simulink library "Sensors_Lib"  (R2018b)
settings: Solver=VariableStepAuto  StartTime=0.0  StopTime=10.0  RelTol=1e-3
undefined symbols (not defined in the file or in its folder): gyro_body_radps, gyro_meas_valid, mag_body_T, mag_meas_valid, photodiodes_A, solar_panel_power_W, sun_meas_ss_deg, sun_meas_valid
libraries: gyroscope_lib x3, magnetometer_lib x3, sensor_bus x1, solar_panels_lib x1, sun_sensor_lib x1
settings Model: Creator=colem  LastModifiedBy=Taylor

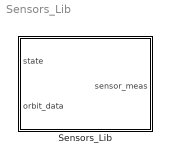
== system Sensors_Lib ==
  Sensors_Lib : Subsystem

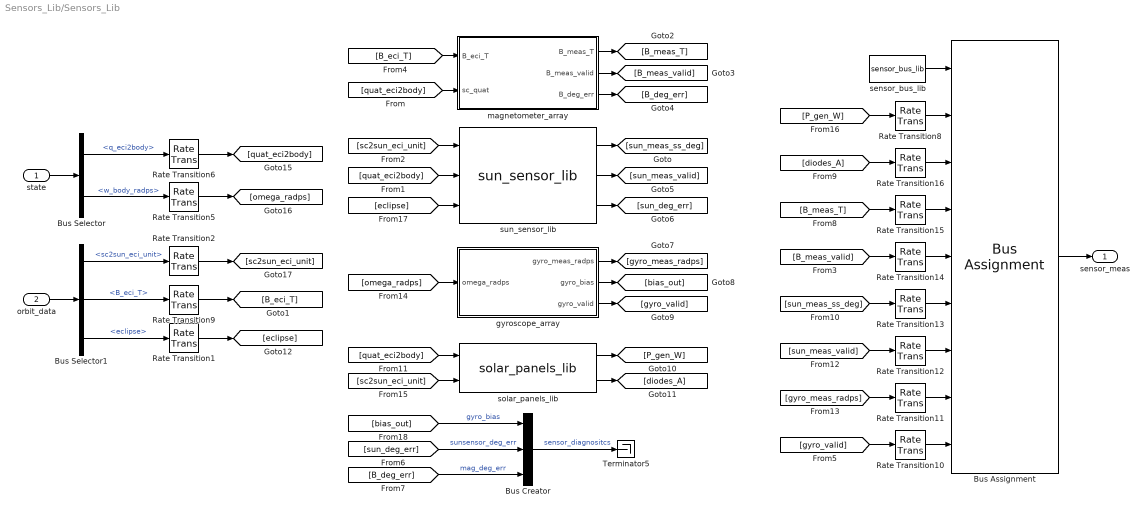
== system Sensors_Lib/Sensors_Lib ==
  state : Inport  OutDataTypeStr=Bus: state
  orbit_data : Inport  Port=2  OutDataTypeStr=Bus: orbit_data
  Bus Assignment : BusAssignment  AssignedSignals=solar_panel_power_W,photodiodes_A,mag_body_T,mag_meas_valid,sun_meas_ss_deg,sun_meas_valid,gyro_body_radps,gyro_meas_valid
  Bus Creator : BusCreator  Inputs=3
  Bus Selector : BusSelector  OutputSignals=q_eci2body,w_body_radps
  Bus Selector1 : BusSelector  OutputSignals=sc2sun_eci_unit,B_eci_T,eclipse
  Rate Transition{1..2,5..6,8..16} (13 alike) : RateTransition  OutPortSampleTime=simParams.sensors.sample_time_s
  Terminator5 : Terminator
  gyroscope_array : Subsystem
  magnetometer_array : Subsystem
  sensor_bus_lib : sensor_bus/sensor_bus_lib  SystemSampleTime=-1
  solar_panels_lib : solar_panels_lib/solar_panels_lib  SystemSampleTime=-1
  "sun_sensor_lib " : sun_sensor_lib/sun_sensor_lib   SystemSampleTime=-1
  sensor_meas : Outport  OutDataTypeStr=Bus: sensor_bus
  wires:
  Bus Selector/2 -> Rate Transition5/1  "<w_body_radps>"
  Bus Assignment/1 -> sensor_meas/1
  [quat_eci2body] -> magnetometer_array/2(sc_quat)
  [quat_eci2body] -> "sun_sensor_lib "/2
  [omega_radps] -> gyroscope_array/1(omega_radps)
  orbit_data/1 -> Bus Selector1/1
  [sc2sun_eci_unit] -> "sun_sensor_lib "/1
  [B_eci_T] -> magnetometer_array/1(B_eci_T)
  sensor_bus_lib/1 -> Bus Assignment/1
  magnetometer_array/1(B_meas_T) -> [B_meas_T]
  magnetometer_array/2(B_meas_valid) -> [B_meas_valid]
  magnetometer_array/3(B_deg_err) -> [B_deg_err]
  "sun_sensor_lib "/1 -> [sun_meas_ss_deg]
  "sun_sensor_lib "/2 -> [sun_meas_valid]
  "sun_sensor_lib "/3 -> [sun_deg_err]
  gyroscope_array/1(gyro_meas_radps) -> [gyro_meas_radps]
  gyroscope_array/2(gyro_bias) -> [bias_out]
  gyroscope_array/3(gyro_valid) -> [gyro_valid]
  Rate Transition5/1 -> [omega_radps]
  Bus Selector/1 -> Rate Transition6/1  "<q_eci2body>"
  Rate Transition6/1 -> [quat_eci2body]
  Bus Selector1/2 -> Rate Transition9/1  "<B_eci_T>"
  Rate Transition9/1 -> [B_eci_T]
  Bus Selector1/1 -> Rate Transition2/1  "<sc2sun_eci_unit>"
  Rate Transition2/1 -> [sc2sun_eci_unit]
  [sc2sun_eci_unit] -> solar_panels_lib/2
  [quat_eci2body] -> solar_panels_lib/1
  solar_panels_lib/1 -> [P_gen_W]
  [B_meas_T] -> Rate Transition15/1
  [P_gen_W] -> Rate Transition8/1
  [B_meas_valid] -> Rate Transition14/1
  [sun_meas_ss_deg] -> Rate Transition13/1
  [sun_meas_valid] -> Rate Transition12/1
  [gyro_meas_radps] -> Rate Transition11/1
  [gyro_valid] -> Rate Transition10/1
  [bias_out] -> Bus Creator/1  "gyro_bias"
  [sun_deg_err] -> Bus Creator/2  "sunsensor_deg_err"
  [B_deg_err] -> Bus Creator/3  "mag_deg_err"
  Bus Creator/1 -> Terminator5/1  "sensor_diagnositcs"
  solar_panels_lib/2 -> [diodes_A]
  Rate Transition10/1 -> Bus Assignment/9
  Rate Transition11/1 -> Bus Assignment/8
  Rate Transition12/1 -> Bus Assignment/7
  Rate Transition13/1 -> Bus Assignment/6
  Rate Transition14/1 -> Bus Assignment/5
  Rate Transition15/1 -> Bus Assignment/4
  Rate Transition8/1 -> Bus Assignment/2
  Rate Transition16/1 -> Bus Assignment/3
  [diodes_A] -> Rate Transition16/1
  state/1 -> Bus Selector/1
  Bus Selector1/3 -> Rate Transition1/1  "<eclipse>"
  Rate Transition1/1 -> [eclipse]
  [eclipse] -> "sun_sensor_lib "/3

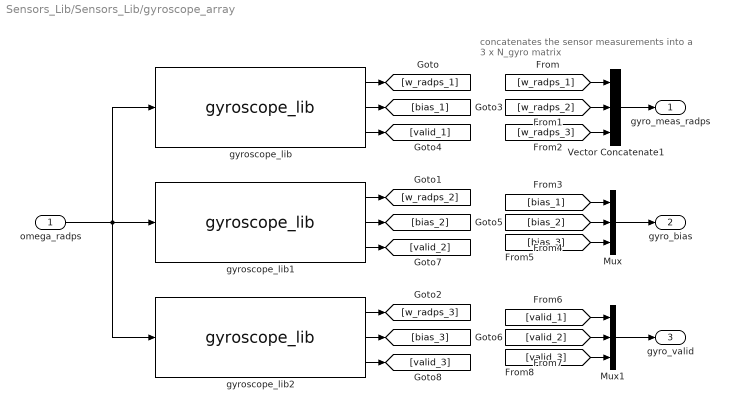
== system Sensors_Lib/Sensors_Lib/gyroscope_array ==
  note: concatenates the sensor measurements
      | into a 3 x N_gyro matrix
  omega_radps : Inport
  Mux : Mux  Inputs=3
  Mux1 : Mux  Inputs=3
  Vector Concatenate1 : Concatenate  NumInputs=3  Mode=Multidimensional array  ConcatenateDimension=2
  gyroscope_lib : gyroscope_lib/gyroscope_lib  id_s=1
  gyroscope_lib1 : gyroscope_lib/gyroscope_lib  id_s=2
  gyroscope_lib2 : gyroscope_lib/gyroscope_lib  id_s=3
  gyro_meas_radps : Outport
  gyro_bias : Outport  Port=2
  gyro_valid : Outport  Port=3
  wires:
  omega_radps/1 -> gyroscope_lib2/1, gyroscope_lib/1, gyroscope_lib1/1
  gyroscope_lib/1 -> [w_radps_1]
  gyroscope_lib1/1 -> [w_radps_2]
  gyroscope_lib2/1 -> [w_radps_3]
  gyroscope_lib/2 -> [bias_1]
  gyroscope_lib/3 -> [valid_1]
  gyroscope_lib1/2 -> [bias_2]
  gyroscope_lib2/2 -> [bias_3]
  gyroscope_lib1/3 -> [valid_2]
  gyroscope_lib2/3 -> [valid_3]
  Vector Concatenate1/1 -> gyro_meas_radps/1
  [w_radps_1] -> Vector Concatenate1/1
  [w_radps_2] -> Vector Concatenate1/2
  [w_radps_3] -> Vector Concatenate1/3
  Mux/1 -> gyro_bias/1
  [bias_1] -> Mux/1
  [bias_2] -> Mux/2
  [bias_3] -> Mux/3
  Mux1/1 -> gyro_valid/1
  [valid_1] -> Mux1/1
  [valid_2] -> Mux1/2
  [valid_3] -> Mux1/3

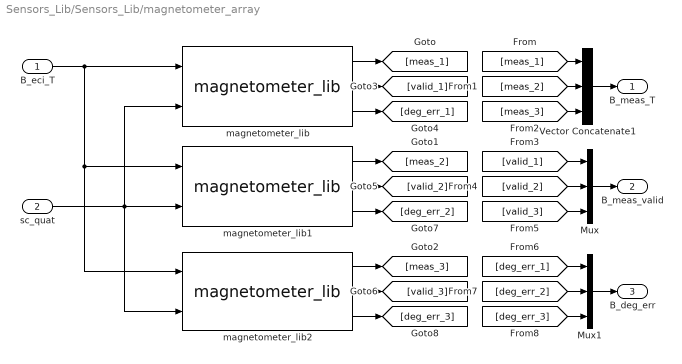
== system Sensors_Lib/Sensors_Lib/magnetometer_array ==
  B_eci_T : Inport
  sc_quat : Inport  Port=2
  Mux : Mux  Inputs=3
  Mux1 : Mux  Inputs=3
  Vector Concatenate1 : Concatenate  NumInputs=3  Mode=Multidimensional array  ConcatenateDimension=2
  magnetometer_lib : magnetometer_lib/magnetometer_lib  id_s=1
  magnetometer_lib1 : magnetometer_lib/magnetometer_lib  id_s=2
  magnetometer_lib2 : magnetometer_lib/magnetometer_lib  id_s=1
  B_meas_T : Outport
  B_meas_valid : Outport  Port=2
  B_deg_err : Outport  Port=3
  wires:
  sc_quat/1 -> magnetometer_lib/2, magnetometer_lib2/2, magnetometer_lib1/2
  B_eci_T/1 -> magnetometer_lib/1, magnetometer_lib2/1, magnetometer_lib1/1
  magnetometer_lib/1 -> [meas_1]
  magnetometer_lib1/1 -> [meas_2]
  magnetometer_lib2/1 -> [meas_3]
  magnetometer_lib/2 -> [valid_1]
  magnetometer_lib/3 -> [deg_err_1]
  magnetometer_lib1/2 -> [valid_2]
  magnetometer_lib2/2 -> [valid_3]
  magnetometer_lib1/3 -> [deg_err_2]
  magnetometer_lib2/3 -> [deg_err_3]
  Vector Concatenate1/1 -> B_meas_T/1
  [meas_1] -> Vector Concatenate1/1
  [meas_2] -> Vector Concatenate1/2
  [meas_3] -> Vector Concatenate1/3
  Mux/1 -> B_meas_valid/1
  [valid_1] -> Mux/1
  [valid_2] -> Mux/2
  [valid_3] -> Mux/3
  Mux1/1 -> B_deg_err/1
  [deg_err_1] -> Mux1/1
  [deg_err_2] -> Mux1/2
  [deg_err_3] -> Mux1/3
